simulink model "SMOKE_detector_857_mod"  (Simulink 7.9)
settings: Solver=ode3  StartTime=0.0  StopTime=inf  RelTol=1e-3
undefined symbols (not defined in the file or in its folder): gray, Rec, SDTV
libraries: visionsinks x3, visionstatistics x2, dspvision x2, visionconversions x1, visiontextngfix x1
(part 1 of 3)
settings Model: Creator=510  LastModifiedBy=room119
settings OptimizationCC: InlineParams=on  InlineInvariantSignals=on  EfficientFloat2IntCast=on  EfficientMapNaN2IntZero=off  OptimizeModelRefInitCode=on  LifeSpan=Inf  SimCompilerOptimization=On  AccelVerboseBuild=on
settings DebuggingCC: UnderspecifiedInitializationDetection=Simplified  ParameterUnderflowMsg=error  ParameterPrecisionLossMsg=none  ParameterTunabilityLossMsg=error  ModelReferenceIOMsg=error  StrictBusMsg=ErrorOnBusTreatedAsVector  NonBusSignalsTreatedAsBus=error
settings HardwareCC: ProdIntDivRoundTo=Zero  ProdHWDeviceType=Generic->32-bit Embedded Processor  TargetHWDeviceType=Generic->32-bit Embedded Processor
settings ModelReferenceCC: EnableParallelModelReferenceBuilds=on
settings SFSimCC: SimParseCustomCode=off  SimBuildMode=sf_make
settings RTWCC: SystemTargetFile=ert.tlc  TemplateMakefile=ert_default_tmf  Description=Embedded Coder  ProcessScript=ert_make_rtw_hook  RTWCompilerOptimization=On
settings CodeAppCC: IgnoreCustomStorageClasses=off
settings ERTTargetCC: CodeReplacementLibrary=ANSI_C  UtilityFuncGeneration=Shared location  MultiwordLength=2048  GenerateSampleERTMain=on  IncludeMdlTerminateFcn=off  SuppressErrorStatus=on  SupportAbsoluteTime=off  MultiInstanceERTCode=on  SupportNonFinite=off  ERTCustomFileTemplate=example_file_process.tlc  PreserveIfCondition=on  ConvertIfToSwitch=off  SuppressUnreachableDefaultCases=off

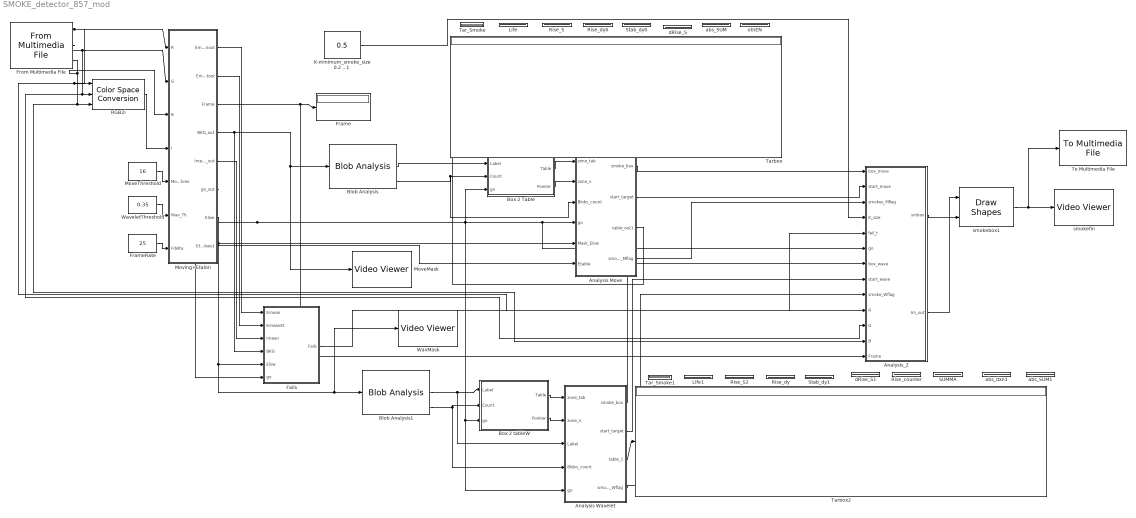
== system SMOKE_detector_857_mod ==
  Analysis Move : MATLAB Function  TreatAsAtomicUnit=on
  Analysis Wavelet : MATLAB Function  TreatAsAtomicUnit=on
  Analysis_2 : MATLAB Function  TreatAsAtomicUnit=on
  Blob Analysis : visionstatistics/Blob Analysis  Tag=vipblks_row_conv  area=off  centroid=off  bBox=on  majorAxis=off  minorAxis=off  angle=off  eccentricity=off  equivDiameterSq=off  extent=off  perimeter=off  maxBlobs=50  warnIfNumBlobsExceeded=on  isCount=on  useMinArea=on  minArea=3  useMaxArea=on  maxArea=900  excludeBorderBlob=off  outDT=double  isOutVarDim=off  isFill=on  fillValues=-1  conn=8  isLabel=on  outputMode=Binary point scaling  outputWordLength=32  outputFracLength=16  firstCoeffMode=Binary point scaling  firstCoeffWordLength=16  firstCoeffFracLength=14  secondCoeffMode=Binary point scaling  secondCoeffWordLength=32  secondCoeffFracLength=16  accumMode=Binary point scaling  accumWordLength=32  accumFracLength=0  prodOutputMode=Binary point scaling  prodOutputWordLength=32  prodOutputFracLength=16  roundingMode=Floor  overflowMode=off
  Blob Analysis1 : visionstatistics/Blob Analysis  Tag=vipblks_row_conv  area=off  centroid=off  bBox=on  majorAxis=off  minorAxis=off  angle=off  eccentricity=off  equivDiameterSq=off  extent=off  perimeter=off  maxBlobs=50  warnIfNumBlobsExceeded=on  isCount=on  useMinArea=on  minArea=3  useMaxArea=on  maxArea=900  excludeBorderBlob=off  outDT=double  isOutVarDim=off  isFill=on  fillValues=-1  conn=8  isLabel=on  outputMode=Binary point scaling  outputWordLength=32  outputFracLength=16  firstCoeffMode=Binary point scaling  firstCoeffWordLength=16  firstCoeffFracLength=14  secondCoeffMode=Binary point scaling  secondCoeffWordLength=32  secondCoeffFracLength=16  accumMode=Binary point scaling  accumWordLength=32  accumFracLength=0  prodOutputMode=Binary point scaling  prodOutputWordLength=32  prodOutputFracLength=16  roundingMode=Floor  overflowMode=off
  Box 2 Table : MATLAB Function  TreatAsAtomicUnit=on
  Box 2 tableW : MATLAB Function  TreatAsAtomicUnit=on
  Fails : MATLAB Function  TreatAsAtomicUnit=on
  Frame : Display
  FrameRate : Constant  Value=25
  From Multimedia File : dspvision/From Multimedia File  inputFilename=D:\SMOKE\VIDEO\std_smoke_videos\gorkogo_red.mp4  loop=on  numPlays=inf  outputStreams=Video only  videoDataType=uint8  audioDataType=int16  inheritSampleTime=on  userDefinedSampleTime=1/30  noAudioOutput=off  isIntensityVideo=off  fourcc=RGB  colorVideoFormat=Separate color signals  outputEOF=off  dataOrg=Column-major  audioFrameSize=800  computeAudioFrameSize=off  outSamplingMode=Sample based
  K-minimum_smoke_size 0.2 .. 1 : Constant  Value=0.5
  Life : Display
  Life1 : Display
  MoveMask : visionsinks/Video Viewer  inputType=Obsolete7b  imagePorts=One multidimensional signal  useColorMap=off  colormapValue=gray(256)  specRange=off  minInputVal=0  maxInputVal=255  FigPos=[-504 758 503 271]  AxisZoom=on  trueSizedOnce=off  OpenAtMdlStart=on
  MoveThreshold : Constant  Value=16
  Moving+Etalon : MATLAB Function  TreatAsAtomicUnit=on
  RGB2i : visionconversions/Color Space  Conversion  conversion=Obsolete  conversionActive=R'G'B' to intensity  wp_str=D65  rec=Rec. 601 (SDTV)  sys=1125/60/2:1  imagePorts=Separate color signals
  Rise_S : Display
  Rise_S2 : Display
  Rise_counter : Display
  Rise_dy : Display
  Rise_dy0 : Display
  SUMMA : Display
  Stab_dy0 : Display
  Stab_dy1 : Display
  Tar_Smoke : Display
  Tar_Smoke1 : Display
  Tarbox : Display
  Tarbox2 : Display
  To Multimedia File : dspvision/To Multimedia File  outputFilename=F:\SMOKE\2109_f.avi  streamSelection=Video only  videoCompressor=None (uncompressed)  audioCompressor=None (uncompressed)  imagePorts=One multidimensional signal  fileType=AVI  audioDatatype=Determine from input data type  fourcc=RGB
  WavMask : visionsinks/Video Viewer  inputType=Obsolete7b  imagePorts=One multidimensional signal  useColorMap=off  colormapValue=gray(256)  specRange=off  minInputVal=0  maxInputVal=255  FigPos=[-502 395 487 280]  AxisZoom=on  trueSizedOnce=off  OpenAtMdlStart=on
  WaveletThreshold : Constant  Value=0.35
  abs_SUM : Display
  abs_SUM1 : Display
  abs_dxn1 : Display
  dRise_S : Display
  dRise_S1 : Display
  otnEN : Display
  smokebox1 : visiontextngfix/Draw Shapes  shape=Rectangles  fill=on  fillClrSource=Specify via dialog  display=User-specified value  intensity=200  color=[255 000 000]  opacity=0.3  viewport=Entire image  antialiasing=off  inType=Obsolete  imagePorts=One multidimensional signal  prodOutputMode=Binary point scaling  prodOutputWordLength=32  prodOutputFracLength=14  memoryMode=Specify word length  memoryWordLength=16  memoryFracLength=14  roundingMode=Floor  overflowMode=off
  smokefin : visionsinks/Video Viewer  inputType=Obsolete7b  imagePorts=One multidimensional signal  useColorMap=off  colormapValue=gray(256)  specRange=off  minInputVal=0  maxInputVal=255  FigPos=[-1023 766 1024 660]  AxisZoom=on  trueSizedOnce=off  OpenAtMdlStart=on
  wires:
  From Multimedia File/1 -> RGB2i/1, Analysis_2/10(R), Moving+Etalon/1(R)
  From Multimedia File/2 -> RGB2i/2, Analysis_2/11(G), Moving+Etalon/2(G)
  From Multimedia File/3 -> RGB2i/3, Analysis_2/12(B), Moving+Etalon/3(B)
  RGB2i/1 -> Moving+Etalon/4(I)
  Moving+Etalon/3(Frame) -> Frame/1, Analysis_2/13(Frame)
  Moving+Etalon/4(BKG_out) -> Fails/4(BKG), Blob Analysis/1, MoveMask/1
  Moving+Etalon/6(go_out) -> Box 2 Table/3(go), Analysis Move/4(go), Analysis_2/6(go), Box 2 tableW/3(go), Analysis Wavelet/5(go), Fails/6(go)
  Moving+Etalon/5(Imean_out) -> Fails/3(Imean)
  Blob Analysis/3 -> Analysis Move/3(Blobs_count), Box 2 Table/2(Count)
  Blob Analysis/2 -> Box 2 Table/1(Label)
  Box 2 Table/2(Pointer) -> Analysis Move/2(zone_n)
  Box 2 tableW/1(Table) -> Analysis Wavelet/1(zone_tab)
  Box 2 tableW/2(Pointer) -> Analysis Wavelet/2(zone_n)
  Blob Analysis1/3 -> Box 2 tableW/2(Count), Analysis Wavelet/4(Blobs_count)
  MoveThreshold/1 -> Moving+Etalon/5(Movthres)
  WaveletThreshold/1 -> Moving+Etalon/6(Wav_Th)
  Analysis Move/3(table_out1) -> Tarbox/1
  Analysis Wavelet/3(table_1) -> Tarbox2/1
  Moving+Etalon/7(Elow) -> Analysis Move/5(Mask_Elow), Fails/5(Elow), Blob Analysis1/1, WavMask/1
  Moving+Etalon/8(Etableout) -> Analysis Move/6(Etable)
  Blob Analysis1/2 -> Box 2 tableW/1(Label), Analysis Wavelet/3(Label)
  Analysis Wavelet/4(smoke_Wflag) -> Analysis_2/9(smoke_Wflag)
  Box 2 Table/1(Table) -> Analysis Move/1(zone_tab)
  FrameRate/1 -> Moving+Etalon/7(Fdelta)
  Moving+Etalon/1(Emeanout) -> Fails/1(Emean)
  Moving+Etalon/2(EmeanEtout) -> Fails/2(EmeanEt)
  Fails/1(Fails) -> Analysis_2/5(fail_t)
  Analysis Wavelet/1(smoke_box) -> Analysis_2/7(box_wave)
  Analysis Move/1(smoke_box) -> Analysis_2/1(box_move)
  Analysis Move/2(start_target) -> Analysis_2/2(start_move)
  Analysis Wavelet/2(start_target) -> Analysis_2/8(start_wave)
  Analysis Move/4(smoke_Mflag) -> Analysis_2/3(smokes_Mflag)
  Analysis_2/1(smbox) -> smokebox1/2
  smokebox1/1 -> smokefin/1, To Multimedia File/1
  K-minimum_smoke_size 0.2 .. 1/1 -> Analysis_2/4(K_size)
  Analysis_2/2(Im_out) -> smokebox1/1

== matlab function Moving+Etalon ==
  data: Emeanout output double; EmeanEtout output double; Frame output double; BKG_out output double; Imean_out output double; R input double; G input double; B input double; I input double; go_out output double; Movthres input double; Wav_Th input double; Elow output double; Etableout output double; Fdelta input double
function [Emeanout, EmeanEtout, Frame, BKG_out,Imean_out,go_out,Elow,Etableout] = func(R,G,B,I,Movthres,Wav_Th,Fdelta)

%% Переменные и Константы

Frame_first=2;

Cell_size=16; % Размер ячейки
LH_frames=80; %Кол-во кадров состояния LH до апдейта 80
Repeat_frames=200; %10/20 Кол-во кадров повторения фона после изменения.
ThRepeat = 7;

BG_H = uint32(8*Cell_size*Cell_size);% 10-Уровень  изменения фона  (Сильное изменение)
BG_L = uint32(4*Cell_size*Cell_size);% 4Уровень фона (Слабое изменение) - Сигнал на обновление
BG_old_l = uint32(5*Cell_size*Cell_size); %4Уровень изменения фона для old (для апдейта не должен быть большим)
BG_old_h = uint32(7*Cell_size*Cell_size);
BG_Move = uint32(Movthres*Cell_size*Cell_size); % Порог для маски движения 16
%Prev_Move = uint32(Prthres*Cell_size*Cell_size); %Порог для маски движения (n-1) 8

E_High = uint8(100);
E_Low = uint8(60);

CoefMult2=10000;%100

[V,H] = size(I);
Vsize = uint16(fix(V/Cell_size)+1);
Hsize = uint16(fix(H/Cell_size)+1);
%2wavelet
segn = fix(V/Cell_size);
segm = fix(H/Cell_size);
%маска сброса зон по отсутсвию движения
reset_wlow_mask=false(Vsize,Hsize);

persistent time
if isempty(time)
    time = uint32(1);
else
    time = time+1;
end
Frame=time;
persistent Fcounter
if isempty(Fcounter)
    Fcounter = uint8(0);
end
persistent KeyFrame
if isempty(KeyFrame)
    KeyFrame = struct('I',uint8(zeros(V,H)),'R',uint8(zeros(V,H)),'G',uint8(zeros(V,H)),'B',uint8(zeros(V,H)));
end;
persistent Frame_old
if isempty(Frame_old)
    Frame_old = struct('I',uint8(zeros(V,H)),'R',uint8(zeros(V,H)),'G',uint8(zeros(V,H)),'B',uint8(zeros(V,H)));
end;
persistent Mask_Color
if isempty(Mask_Color)
    Mask_Color = false(V,H);
end
persistent Imean
if isempty(Imean)
    Imean = uint8(0);
end
persistent Imean_Prev
if isempty(Imean_Prev)
    Imean_Prev= uint8(0);
end
persistent W_flag_low
if isempty(W_flag_low)
    W_flag_low=false(Vsize,Hsize);
end;
persistent delta
if isempty(delta)
    delta=zeros(Vsize,Hsize);
end;
persistent Etable
if isempty (Etable)
    Etable=int32(zeros(Vsize,Hsize));
end
persistent EtableEt
if isempty (EtableEt)
    EtableEt=int32(zeros(Vsize,Hsize));
end
persistent Emean
if isempty(Emean)
    Emean=int32(0);
end
persistent EmeanEt
if isempty(EmeanEt)
    EmeanEt=int32(0);
end
persistent txins
if isempty(txins)
    txins = vision.TextInserter('Text', '%4d', 'Location',  [0 4], ...
        'Color', [0 0 0], 'FontSize', 7);
end
persistent Imtab
if isempty(Imtab)
    Imtab=uint8(zeros(V,H,1));
end
Imseg1 =uint8(zeros(Cell_size,Cell_size));

BKG_out=false(Vsize,Hsize);
ws=Cell_size/2;
LL1=zeros(ws,ws);
LH1=zeros(ws,ws);
HL1=zeros(ws,ws);
HH1=zeros(ws,ws);
LL2=zeros(ws,ws);
LH2=zeros(ws,ws);
HL2=zeros(ws,ws);
HH2=zeros(ws,ws);
Id=zeros(V,H);
Ikfd=zeros(V,H);
%
TCell=struct('Sub_EtalonR',uint32(0),'Sub_EtalonG',uint32(0),'Sub_EtalonB',uint32(0),...
    'Sub_EtalonI',uint32(0),'Sub_PrevR',uint32(0),'Sub_PrevG',uint32(0),'Sub_PrevB',uint32(0),...
    'Sub_PrevI',uint32(0),'Rewrite',false,'LH_Counter',uint8(0), 'Repeat_Counter',uint8(0),'MoveMask',false,'Imean_Rewrite',uint8(0));%
persistent Cells
if isempty(Cells)
    Cells = repmat(TCell,Vsize,Hsize);
end
%Etalon_out =uint8(zeros(V,H));
coder.extrinsic('dwt2','im2double');
%% MAIN
% Запись первого кадра
if time == Frame_first
    KeyFrame.R=R;
    KeyFrame.G=G;
    KeyFrame.B=B;
    KeyFrame.I=I;
    Frame_old.R=uint8(R);
    Frame_old.G=uint8(G);
    Frame_old.B=uint8(B);
    Frame_old.I=uint8(I);
    Isum=uint32(sum(I(:)));
    Imean=uint8(Isum/(V*H));
end
%Счетчик N-го кадра
if (Fcounter<fix(Fdelta/2))&&(time > Frame_first)%849
    Fcounter=Fcounter+1;
else
    Fcounter=uint8(1);
end;

go_out=0;
% Если кадр кратен N
if (Fcounter==1) && (time > Frame_first)
    Isum=uint32(0);
    Isum_KF=uint32(0);
    go_out=1;
    for i=1:V
        for j=1:H
            Isum= Isum+uint32(I(i,j));
            Isum_KF=Isum_KF+uint32(KeyFrame.I(i,j));
            %% Маска по цвету
            Mask_Color(i,j)=false;
            % Sum_delta= abs(int16(R(i,j))-int16(G(i,j))) + abs(int16(R(i,j))-int16(B(i,j))) + abs(int16(B(i,j))-int16(G(i,j)));
            % Поиск максимума и минимума
            if (R(i,j)>=G(i,j)) && (R(i,j)>=B(i,j))
                maxi=R(i,j);
                if G(i,j)>B(i,j)
                    mini=B(i,j);
                    mean=G(i,j);
                else
                    mini=G(i,j);
                    mean=B(i,j);
                end;
            else
                if G(i,j)>B(i,j)
                    maxi=G(i,j);
                    if R(i,j)>B(i,j)
                        mini=B(i,j);
                        mean=R(i,j);
                    else
                        mini=R(i,j);
                        mean=B(i,j);
                    end;
                else
                    maxi=B(i,j);
                    if R(i,j)>G(i,j)
                        mini=G(i,j);
                        mean=R(i,j);
                    else
                        mini=R(i,j);
                        mean=G(i,j);
                    end;
                end;
            end;
            %Вычисление дельт
            delta_max=maxi-mini;
            delta_left=mean-mini;
            delta_right=maxi-mean;
            if delta_left>delta_right
                delta_min=delta_right;
            else
                delta_min=delta_left;
            end;
            % Условие Цветности
            if delta_max>86
                Mask_Color(i,j)=true;
            else
                if delta_max>50
                    if (delta_max/maxi)>0.5
                        Mask_Color(i,j)=true;
                    end
                    if (delta_max/delta_min) >7
                        Mask_Color(i,j)=true;
                    end
                end
            end
            
            %% Рачет фона для Cells
            n=uint16(fix((i-1)/Cell_size)+1);
            m=uint16(fix((j-1)/Cell_size)+1);
            if n > Vsize
                n=uint16(Vsize);
            end
            if m > Hsize
                m=uint16(Hsize);
            end
            if  ~(Mask_Color(i,j))
                % Сравнение с эталоном
                Cells(n,m).Sub_EtalonR=Cells(n,m).Sub_EtalonR+uint32(abs(int16(KeyFrame.R(i,j))-int16(R(i,j))));
                Cells(n,m).Sub_EtalonG=Cells(n,m).Sub_EtalonG+uint32(abs(int16(KeyFrame.G(i,j))-int16(G(i,j))));
                Cells(n,m).Sub_EtalonB=Cells(n,m).Sub_EtalonB+uint32(abs(int16(KeyFrame.B(i,j))-int16(B(i,j))));
                Cells(n,m).Sub_EtalonI=Cells(n,m).Sub_EtalonI+uint32(abs( int16(KeyFrame.I(i,j))-int16(I(i,j))));
                % Сравнение с N-1 кадром
                Cells(n,m).Sub_PrevR=Cells(n,m).Sub_PrevR+uint32(abs(int16(Frame_old.R(i,j))-int16(R(i,j))));
                Cells(n,m).Sub_PrevG=Cells(n,m).Sub_PrevG+uint32(abs(int16(Frame_old.G(i,j))-int16(G(i,j))));
                Cells(n,m).Sub_PrevB=Cells(n,m).Sub_PrevB+uint32(abs(int16(Frame_old.B(i,j))-int16(B(i,j))));
                Cells(n,m).Sub_PrevI=Cells(n,m).Sub_PrevI+uint32(abs( int16(Frame_old.I(i,j))-int16(I(i,j))));
            end
            Frame_old.R(i,j)=R(i,j);
            Frame_old.G(i,j)=G(i,j);
            Frame_old.B(i,j)=B(i,j);
            Frame_old.I(i,j)=I(i,j);
        end
    end
    % Средняя яркость текущего кадра и эталонного
    Imean=uint8(Isum/(V*H));
    %% Анализ фона в ячейках
    for n=1:Vsize
        for m=1:Hsize
            if (abs(int16(Imean_Prev)-int16(Imean))>30)
                Cells(n,m).Rewrite=true;
            else
                %% Маска движения
                if  (Cells(n,m).Sub_EtalonR>=BG_Move) ||  (Cells(n,m).Sub_EtalonG>=BG_Move) ...
                        ||(Cells(n,m).Sub_EtalonB>=BG_Move) || (Cells(n,m).Sub_EtalonI>=BG_Move)
                    %Маска Движения
                    Cells(n,m).MoveMask=true;
                else
                    Cells(n,m).MoveMask=false;
                end;
                %% Проверка межкадровой повторяемости в зонах (корректор выходных масок)
                if (Cells(n,m).Repeat_Counter > ThRepeat)
                    Cells(n,m).MoveMask=false;
                    % МАТРИЦА ФЛАГОВ СБРОСА ЗОН в ВЕВЛЕТ-маске
                    reset_wlow_mask(n,m)=true;
                else
                    reset_wlow_mask(n,m)=false;
                end;
                % Адаптация порога для роста счетчика Repeat
                if (Etable(n,m)>=E_High)
                    BG_old=BG_old_h;
                else
                    BG_old=BG_old_l;
                end
                %% Для Обновления
                % Условие 1 - Если зона на текущем кадра сильно отличается от эталона
                if  ((Cells(n,m).Sub_EtalonR>=BG_H) ||  (Cells(n,m).Sub_EtalonG>=BG_H) ...
                        ||(Cells(n,m).Sub_EtalonB>=BG_H) || (Cells(n,m).Sub_EtalonI>=BG_H))%&&Cells(n,m).MoveMask==false);%815  
                    Cells(n,m).LH_Counter=uint8(0);
                    % 1.1 Нет изменений между соседними кадрами + счетчик таких событий
                    if (((Cells(n,m).Sub_PrevB<BG_old) && (Cells(n,m).Sub_PrevI<BG_old)) ...
                            || ((Cells(n,m).Sub_PrevG<BG_old) && (Cells(n,m).Sub_PrevI<BG_old))...
                            ||((Cells(n,m).Sub_PrevR<BG_old) && (Cells(n,m).Sub_PrevI<BG_old)))
                        % Счетчик повторяемости соседних кадров
                        Cells(n,m).Repeat_Counter=Cells(n,m).Repeat_Counter+1;
                        %Условия для обновления (Rewrite) 
                        if (Etable(n,m) < E_Low)
                            if(Cells(n,m).Repeat_Counter >= (Repeat_frames*3))
                                Cells(n,m).Rewrite=true;
                            end
                        elseif (Etable(n,m) < E_High)
                            if(Cells(n,m).Repeat_Counter >= (Repeat_frames*2))
                                Cells(n,m).Rewrite=true;
                            end
                        else
                            if (Cells(n,m).Repeat_Counter >= Repeat_frames)
                                Cells(n,m).Rewrite=true;
                            end
                        end
                    else
                        Cells(n,m).Repeat_Counter=uint8(0);
                    end
                % Условие 2 - Если зона на текущем кадре совсем слабо отличается от эталона (для наступления сумерек или  рассвета - плавного)
                elseif (Cells(n,m).Sub_EtalonR<BG_L) && (Cells(n,m).Sub_EtalonG<BG_L) &&  (Cells(n,m).Sub_EtalonB<BG_L) && (Cells(n,m).Sub_EtalonI<BG_L) %Нет изменений ни в одном канале
                    Cells(n,m).Rewrite=true;% ОБНОВЛЕНИЕ
                % Условие 3 - Если не У1 и не У2, те когда среднее изменение от эталона = от BG_L до BG_H (используется счетчик LH_COUNTER)
                else
                    Cells(n,m).LH_Counter = Cells(n,m).LH_Counter+1;
                    if Cells(n,m).LH_Counter >=LH_frames
                        Cells(n,m).Rewrite=true; % ОБНОВЛЕНИЕ
                    end
                end;
            end;
            %% Перезапись эталона по Rewrite или резкому изменению яркости кадра
            Cells(n,m).Sub_EtalonR = uint32(0);
            Cells(n,m).Sub_EtalonG = uint32(0);
            Cells(n,m).Sub_EtalonB = uint32(0);
            Cells(n,m).Sub_EtalonI = uint32(0);
            Cells(n,m).Sub_PrevR = uint32(0);
            Cells(n,m).Sub_PrevG = uint32(0);
            Cells(n,m).Sub_PrevB = uint32(0);
            Cells(n,m).Sub_PrevI = uint32(0);
            
            if Cells(n,m).Rewrite
                Cells(n,m).Rewrite=false;
                Cells(n,m).LH_Counter=uint8(0);
                Cells(n,m).Repeat_Counter=uint8(0);
                Cells(n,m).Imean_Rewrite=Imean;%
                
                xo=(m-1)*Cell_size+1;
                xn=m*Cell_size;
                yo=(n-1)*Cell_size+1;
                yn=n*Cell_size;
                if yn>V
                    yn=uint16(V);
                end;
                if xn>H
                    xn=uint16(H);
                end;

                for  i=yo:yn
                    for j=xo:xn
                        KeyFrame.R(i,j)=R(i,j);
                        KeyFrame.G(i,j)=G(i,j);
                        KeyFrame.B(i,j)=B(i,j);
                        KeyFrame.I(i,j)=I(i,j);
                    end;
                end;
            end;
        end
    end
    
    %%  WAVELET
    Id=im2double(I);
    Ikfd=im2double(KeyFrame.I);
    
    if  (time > Frame_first)
        for i=1:segn
            for j=1:segm
                %%
                % текущий кадр
                Imseg = Id((i-1)*Cell_size+1:i*Cell_size,(j-1)*Cell_size+1:j*Cell_size);
                [LL1,LH1,HL1,HH1]=dwt2(Imseg,'haar');
                Esum=0;
                Esum1=0;
                [wn,wm]=size(HH1);
                % эталонный кадр
                ImsegEt = Ikfd((i-1)*Cell_size+1:i*Cell_size,(j-1)*Cell_size+1:j*Cell_size);
                [LL2,LH2,HL2,HH2]=dwt2(ImsegEt,'haar');
                EsumEt=0;
                
                % суммирование в зоне
                for y=1:wn
                    for x=1:wm
                        % сумма по всем коэф.
                        E=abs((HL1(x,y)^2)+(LH1(x,y)^2)+(HH1(x,y)^2));
                        Esum=Esum+E;
                        Eet=abs((LH2(x,y)^2)+(HL2(x,y)^2)+(HH2(x,y)^2));
                        EsumEt=EsumEt+Eet;
                    end
                end
                
                Esum=(CoefMult2*Esum)+1;
                EsumEt=(CoefMult2*EsumEt)+1;
                Etable(i,j)=int32(Esum/100);
                EtableEt(i,j)=int32(EsumEt/100);
                Delta_E_low=((EsumEt-Esum)/EsumEt);
                
                if (Delta_E_low > Wav_Th) && (~reset_wlow_mask(i,j)) %Падение энергии в сегменте и 582:сброс по отсутсвию движения
                    W_flag_low(i,j)=true;
                else
                    W_flag_low(i,j)=false;
                end;
            end
        end
    end
end

%% Вывод данных
if time>=20
    %Рисование Movepic
    for i=1:segn
        for j=1:segm
            
            if Cells(i,j).MoveMask==0 %W_flag_low(i,j)
                Imseg1 =uint8(zeros(Cell_size,Cell_size));
            else
                Imseg1 = I((i-1)*Cell_size+1:i*Cell_size,(j-1)*Cell_size+1:j*Cell_size);
                %Imseg1 = step(txins,Imseg1, Etable(i,j));
            end
            
            Imtab((i-1)*Cell_size+1:i*Cell_size,(j-1)*Cell_size+1:j*Cell_size) = Imseg1;
        end
    end
end

% 845 Рисование цветовой маски и средней Е
Etablesum=int32(0); %845
EtablesumEt=int32(0);%845

for n=1:Vsize
    for m=1:Hsize
        BKG_out(n,m)=Cells(n,m).MoveMask;
        Etablesum=Etablesum+Etable(n,m); %845
        EtablesumEt=EtablesumEt+EtableEt(n,m); %845
    end;
end;

Emean=(Etablesum/int32(Vsize*Hsize)); %845
Emeanout=Emean;                 %845
EmeanEt=(EtablesumEt/int32(Vsize*Hsize)); %845
EmeanEtout=EmeanEt;             %845

Imean_Prev=Imean;
Imean_out=Imean;
Elow=W_flag_low;
Etableout=Etable;
